simulink model "ASE_372K_FinalProj_AttD"  (R2018b)
settings: Solver=VariableStepAuto  StartTime=0.0  StopTime=5370  FixedStep=100  RelTol=1e-3
libraries: simulink x3, sharedtransform x3
settings Model: SimulationMode=accelerator  Creator=kenda  LastModifiedBy=kenda

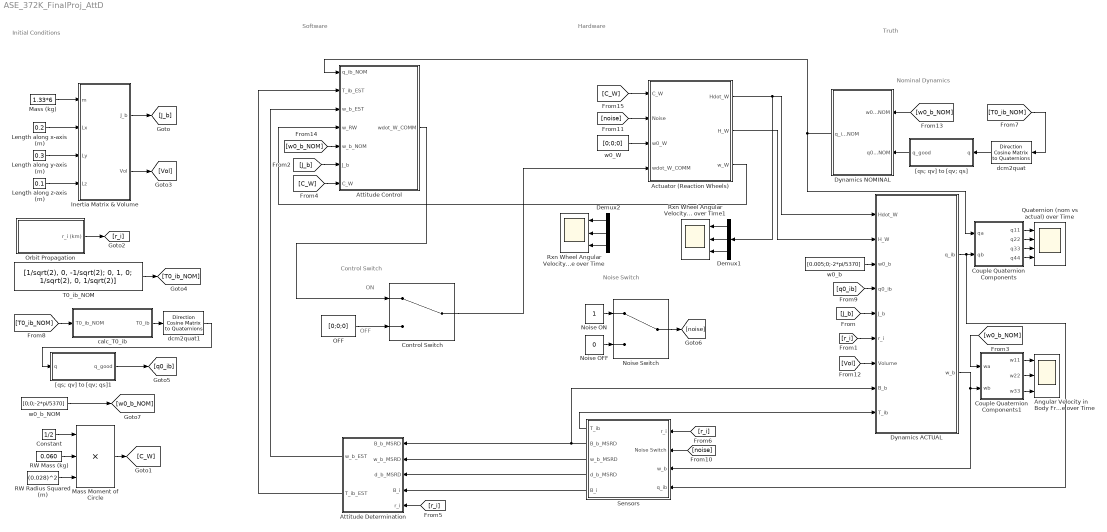
== system ASE_372K_FinalProj_AttD ==
  note: ON
  note: Truth
  note: Software
  note: Hardware
  note: Noise Switch
  note: OFF
  note: Control Switch
  note: Initial Conditions
  note: Nominal Dynamics
  Actuator (Reaction Wheels) : Subsystem
  Angular Velocity in Body Frame over Time : Scope  NumInputPorts=3
  Attitude Control : Subsystem
  Attitude Determination : Subsystem
  Constant : Constant  Value=1/2
  Control Switch : ManualSwitch
  Couple Quaternion Components : MATLAB Function  TreatAsAtomicUnit=on
  Couple Quaternion Components1 : MATLAB Function  TreatAsAtomicUnit=on
  Demux1 : Demux  Outputs=3
  Demux2 : Demux  Outputs=3
  Dynamics ACTUAL : Subsystem
  Dynamics NOMINAL : Subsystem
  Inertia Matrix & Volume : MATLAB Function  TreatAsAtomicUnit=on
  Length along x-axis (m) : Constant  Value=0.2
  Length along y-axis (m) : Constant  Value=0.3
  Length along z-axis (m) : Constant  Value=0.1
  Mass (kg) : Constant  Value=1.33*6
  Mass Moment of Circle : Product  Inputs=3
  Noise OFF : Constant  Value=0
  Noise ON : Constant
  Noise Switch : ManualSwitch
  OFF : Constant  Value=[0;0;0]
  Orbit Propagation : Subsystem
  Quaternion (nom vs actual) over Time : Scope  NumInputPorts=4
  RW Mass (kg) : Constant  Value=0.060
  RW Radius Squared (m) : Constant  Value=(0.028)^2
  Rxn Wheel Angular Velocity in Body Frame over Time : Scope  NumInputPorts=3
  Rxn Wheel Angular Velocity in Body Frame over Time1 : Scope  NumInputPorts=3
  Sensors : Subsystem
  T0_ib_NOM : Constant  Value=[1/sqrt(2), 0, -1/sqrt(2); 0, 1, 0; 1/sqrt(2), 0, 1/sqrt(2)]
  "[qs; qv] to [qv; qs]" : MATLAB Function  TreatAsAtomicUnit=on
  "[qs; qv] to [qv; qs]1" : MATLAB Function  TreatAsAtomicUnit=on
  calc_T0_ib : MATLAB Function  TreatAsAtomicUnit=on
  dcm2quat : sharedtransform/Direction Cosine Matrix  to Quaternions  aMode=0  action=None  tolerance=eps(2)
      settings: SourceProductName=Aerospace Blockset  SourceProductBaseCode=AE
  dcm2quat1 : sharedtransform/Direction Cosine Matrix  to Quaternions  aMode=0  action=None  tolerance=eps(2)
      settings: SourceProductName=Aerospace Blockset  SourceProductBaseCode=AE
  w0_W : Constant  Value=[0;0;0]
  w0_b : Constant  Value=[0.005;0;-2*pi/5370]
  w0_b_NOM : Constant  Value=[0;0;-2*pi/5370]
  wires:
  Dynamics ACTUAL/2(w_b) -> Couple Quaternion Components1/2(wb), Sensors/3(w_b)
  w0_W/1 -> Actuator (Reaction Wheels)/3(w0_W)
  w0_b/1 -> Dynamics ACTUAL/3(w0_b)
  [J_b] -> Dynamics ACTUAL/5(J_b)
  Actuator (Reaction Wheels)/2(H_W) -> Dynamics ACTUAL/2(H_W)
  [q0_ib] -> Dynamics ACTUAL/4(q0_ib)
  [C_W] -> Actuator (Reaction Wheels)/1(C_W)
  Actuator (Reaction Wheels)/1(Hdot_W) -> Demux1/1, Dynamics ACTUAL/1(Hdot_W)
  Sensors/3(w_b_MSRD) -> Attitude Determination/2(w_b_MSRD)
  Sensors/2(B_b_MSRD) -> Dynamics ACTUAL/8(B_b), Attitude Determination/1(B_b_MSRD)
  Dynamics ACTUAL/1(q_ib) -> Sensors/4(q_ib), Couple Quaternion Components/2(qb)
  [r_i] -> Attitude Determination/5(r_i)
  [r_i] -> Sensors/1(r_i)
  Actuator (Reaction Wheels)/3(w_W) -> Attitude Control/4(w_RW)
  Attitude Determination/1(w_b_EST) -> Attitude Control/3(w_b_EST)
  Attitude Determination/2(T_ib_EST) -> Attitude Control/2(T_ib_EST)
  Dynamics NOMINAL/1(q_ib_NOM) -> Couple Quaternion Components/1(qa), Attitude Control/1(q_ib_NOM)
  Attitude Control/1(wdot_W_COMM) -> Control Switch/1
  [J_b] -> Attitude Control/6(J_b)
  dcm2quat/1 -> "[qs; qv] to [qv; qs]"/1(q)
  [T0_ib_NOM] -> dcm2quat/1
  [T0_ib_NOM] -> calc_T0_ib/1(T0_ib_NOM)
  T0_ib_NOM/1 -> [T0_ib_NOM]
  dcm2quat1/1 -> "[qs; qv] to [qv; qs]1"/1(q)
  calc_T0_ib/1(T0_ib) -> dcm2quat1/1
  "[qs; qv] to [qv; qs]1"/1(q_good) -> [q0_ib]
  "[qs; qv] to [qv; qs]"/1(q_good) -> Dynamics NOMINAL/2(q0_ib_NOM)
  Noise Switch/1 -> [noise]
  Noise ON/1 -> Noise Switch/1
  Noise OFF/1 -> Noise Switch/2
  [noise] -> Sensors/2(Noise Switch)
  [noise] -> Actuator (Reaction Wheels)/2("Noise ")
  Control Switch/1 -> Actuator (Reaction Wheels)/4(wdot_W_COMM)
  Demux2/2 -> Rxn Wheel Angular Velocity in Body Frame over Time/2
  Demux2/1 -> Rxn Wheel Angular Velocity in Body Frame over Time/1
  Demux2/3 -> Rxn Wheel Angular Velocity in Body Frame over Time/3
  Orbit Propagation/1(r_i (km)) -> [r_i]
  [r_i] -> Dynamics ACTUAL/6(r_i)
  Mass (kg)/1 -> Inertia Matrix & Volume/1(m)
  Sensors/4(d_b_MSRD) -> Attitude Determination/3(d_b_MSRD)
  Sensors/5(B_i) -> Attitude Determination/4(B_i)
  Sensors/1(T_ib) -> Dynamics ACTUAL/9(T_ib)
  Inertia Matrix & Volume/2(Vol) -> [Vol]
  [Vol] -> Dynamics ACTUAL/7(Volume)
  w0_b_NOM/1 -> [w0_b_NOM]
  [w0_b_NOM] -> Dynamics NOMINAL/1(w0_b_NOM)
  [w0_b_NOM] -> Attitude Control/5(w_b_NOM)
  OFF/1 -> Control Switch/2
  [C_W] -> Attitude Control/7(C_W)
  Inertia Matrix & Volume/1(J_b) -> [J_b]
  Length along y-axis (m)/1 -> Inertia Matrix & Volume/3(Ly)
  Length along x-axis (m)/1 -> Inertia Matrix & Volume/2(Lx)
  Length along z-axis (m)/1 -> Inertia Matrix & Volume/4(Lz)
  Constant/1 -> Mass Moment of Circle/1
  RW Mass (kg)/1 -> Mass Moment of Circle/2
  RW Radius Squared (m)/1 -> Mass Moment of Circle/3
  Mass Moment of Circle/1 -> [C_W]
  Couple Quaternion Components/1(q11) -> Quaternion (nom vs actual) over Time/1
  Couple Quaternion Components/2(q22) -> Quaternion (nom vs actual) over Time/2
  Couple Quaternion Components/3(q33) -> Quaternion (nom vs actual) over Time/3
  Couple Quaternion Components/4(q44) -> Quaternion (nom vs actual) over Time/4
  Couple Quaternion Components1/1(w11) -> Angular Velocity in Body Frame over Time/1
  Couple Quaternion Components1/2(w22) -> Angular Velocity in Body Frame over Time/2
  Couple Quaternion Components1/3(w33) -> Angular Velocity in Body Frame over Time/3
  [w0_b_NOM] -> Couple Quaternion Components1/1(wa)
  Demux1/2 -> Rxn Wheel Angular Velocity in Body Frame over Time1/2
  Demux1/3 -> Rxn Wheel Angular Velocity in Body Frame over Time1/3
  Demux1/1 -> Rxn Wheel Angular Velocity in Body Frame over Time1/1

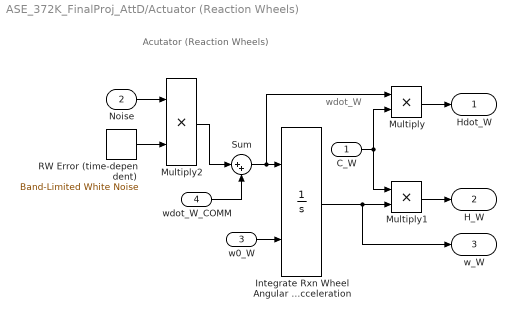
== system ASE_372K_FinalProj_AttD/Actuator (Reaction Wheels) ==
  note: wdot_W
  note: Acutator (Reaction Wheels)
  C_W : Inport
  "Noise " : Inport  Port=2
  w0_W : Inport  Port=3
  wdot_W_COMM : Inport  Port=4
  Integrate Rxn Wheel Angular Acceleration : Integrator  InitialConditionSource=external  ContinuousStateAttributes='ang_vel'
  Multiply : Product
  Multiply1 : Product
  Multiply2 : Product
  RW Error (time-dependent) : simulink/Sources/Band-Limited White Noise  Cov=1e-6*[1;1;1]  Ts=1  seed=[23341]
  Sum : Sum  Inputs=|++
  Hdot_W : Outport
  H_W : Outport  Port=2
  w_W : Outport  Port=3
  wires:
  w0_W/1 -> Integrate Rxn Wheel Angular Acceleration/2
  Sum/1 -> Multiply/1, Integrate Rxn Wheel Angular Acceleration/1
  RW Error (time-dependent)/1 -> Multiply2/2
  Multiply/1 -> Hdot_W/1
  C_W/1 -> Multiply1/1, Multiply/2
  Integrate Rxn Wheel Angular Acceleration/1 -> w_W/1, Multiply1/2
  Multiply1/1 -> H_W/1
  "Noise "/1 -> Multiply2/1
  Multiply2/1 -> Sum/1
  wdot_W_COMM/1 -> Sum/2

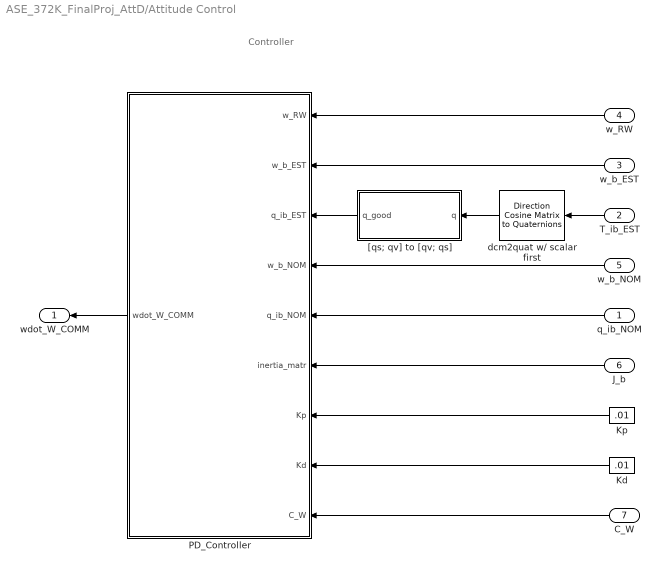
== system ASE_372K_FinalProj_AttD/Attitude Control ==
  note: Controller
  q_ib_NOM : Inport
  T_ib_EST : Inport  Port=2
  w_b_EST : Inport  Port=3
  w_RW : Inport  Port=4
  w_b_NOM : Inport  Port=5
  J_b : Inport  Port=6
  C_W : Inport  Port=7
  Kd : Constant  Value=.01
  Kp : Constant  Value=.01
  PD_Controller : MATLAB Function  TreatAsAtomicUnit=on
  "[qs; qv] to [qv; qs]" : MATLAB Function  TreatAsAtomicUnit=on
  dcm2quat w/ scalar first : sharedtransform/Direction Cosine Matrix  to Quaternions  aMode=0  action=None  tolerance=eps(2)
      settings: SourceProductName=Aerospace Blockset  SourceProductBaseCode=AE
  wdot_W_COMM : Outport
  wires:
  Kd/1 -> PD_Controller/8(Kd)
  w_b_NOM/1 -> PD_Controller/4(w_b_NOM)
  Kp/1 -> PD_Controller/7(Kp)
  J_b/1 -> PD_Controller/6(inertia_matr)
  PD_Controller/1(wdot_W_COMM) -> wdot_W_COMM/1
  C_W/1 -> PD_Controller/9(C_W)
  w_RW/1 -> PD_Controller/1(w_RW)
  w_b_EST/1 -> PD_Controller/2(w_b_EST)
  q_ib_NOM/1 -> PD_Controller/5(q_ib_NOM)
  T_ib_EST/1 -> dcm2quat w/ scalar first/1
  dcm2quat w/ scalar first/1 -> "[qs; qv] to [qv; qs]"/1(q)
  "[qs; qv] to [qv; qs]"/1(q_good) -> PD_Controller/3(q_ib_EST)

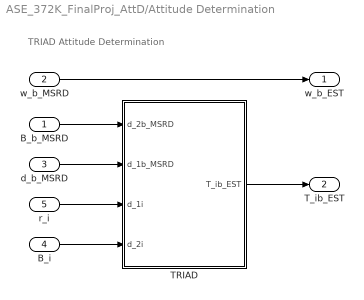
== system ASE_372K_FinalProj_AttD/Attitude Determination ==
  note: TRIAD Attitude Determination
  B_b_MSRD : Inport
  w_b_MSRD : Inport  Port=2
  d_b_MSRD : Inport  Port=3
  B_i : Inport  Port=4
  r_i : Inport  Port=5
  TRIAD : MATLAB Function  TreatAsAtomicUnit=on
  w_b_EST : Outport
  T_ib_EST : Outport  Port=2
  wires:
  w_b_MSRD/1 -> w_b_EST/1
  d_b_MSRD/1 -> TRIAD/2(d_1b_MSRD)
  B_b_MSRD/1 -> TRIAD/1(d_2b_MSRD)
  r_i/1 -> TRIAD/3(d_1i)
  B_i/1 -> TRIAD/4(d_2i)
  TRIAD/1(T_ib_EST) -> T_ib_EST/1

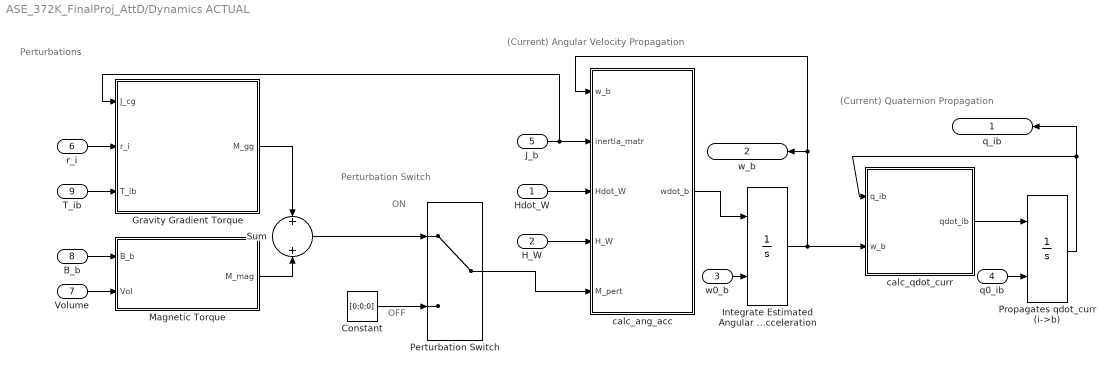
== system ASE_372K_FinalProj_AttD/Dynamics ACTUAL ==
  note: ON
  note: Perturbations
  note: (Current) Angular Velocity Propagation
  note: (Current) Quaternion Propagation
  note: OFF
  note: Perturbation Switch
  Hdot_W : Inport
  H_W : Inport  Port=2
  w0_b : Inport  Port=3
  q0_ib : Inport  Port=4
  J_b : Inport  Port=5
  r_i : Inport  Port=6
  Volume : Inport  Port=7
  B_b : Inport  Port=8
  T_ib : Inport  Port=9
  Constant : Constant  Value=[0;0;0]
  Gravity Gradient Torque : MATLAB Function  TreatAsAtomicUnit=on
  Integrate Estimated Angular Acceleration : Integrator  InitialConditionSource=external  ContinuousStateAttributes='ang_vel'
  Magnetic Torque : MATLAB Function  TreatAsAtomicUnit=on
  Perturbation Switch : ManualSwitch
  Propagates qdot_curr (i->b) : Integrator  InitialConditionSource=external  ContinuousStateAttributes='qdot_curr'
  Sum : Sum  Inputs=+||+
  calc_ang_acc : MATLAB Function  TreatAsAtomicUnit=on
  calc_qdot_curr : MATLAB Function  TreatAsAtomicUnit=on
  q_ib : Outport
  w_b : Outport  Port=2
  wires:
  w0_b/1 -> Integrate Estimated Angular Acceleration/2
  Integrate Estimated Angular Acceleration/1 -> w_b/1, calc_ang_acc/1(w_b), calc_qdot_curr/2(w_b)
  q0_ib/1 -> Propagates qdot_curr (i->b)/2
  calc_qdot_curr/1(qdot_ib) -> Propagates qdot_curr (i->b)/1
  Propagates qdot_curr (i->b)/1 -> calc_qdot_curr/1(q_ib), q_ib/1
  H_W/1 -> calc_ang_acc/4(H_W)
  Hdot_W/1 -> calc_ang_acc/3(Hdot_W)
  calc_ang_acc/1(wdot_b) -> Integrate Estimated Angular Acceleration/1
  r_i/1 -> Gravity Gradient Torque/2(r_i)
  J_b/1 -> Gravity Gradient Torque/1(J_cg), calc_ang_acc/2(inertia_matr)
  B_b/1 -> Magnetic Torque/1(B_b)
  Magnetic Torque/1(M_mag) -> Sum/2
  T_ib/1 -> Gravity Gradient Torque/3(T_ib)
  Gravity Gradient Torque/1(M_gg) -> Sum/1
  Volume/1 -> Magnetic Torque/2(Vol)
  Sum/1 -> Perturbation Switch/1
  Constant/1 -> Perturbation Switch/2
  Perturbation Switch/1 -> calc_ang_acc/5(M_pert)

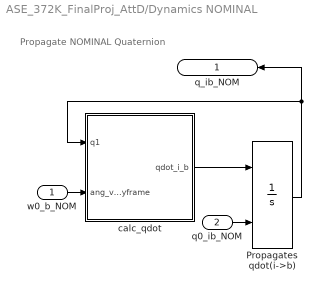
== system ASE_372K_FinalProj_AttD/Dynamics NOMINAL ==
  note: Propagate NOMINAL Quaternion
  w0_b_NOM : Inport
  q0_ib_NOM : Inport  Port=2
  Propagates qdot(i->b) : Integrator  InitialConditionSource=external  ContinuousStateAttributes='qdot_curr'
  calc_qdot : MATLAB Function  TreatAsAtomicUnit=on
  q_ib_NOM : Outport
  wires:
  q0_ib_NOM/1 -> Propagates qdot(i->b)/2
  Propagates qdot(i->b)/1 -> q_ib_NOM/1, calc_qdot/1(q1)
  calc_qdot/1(qdot_i_b) -> Propagates qdot(i->b)/1
  w0_b_NOM/1 -> calc_qdot/2(ang_vel_bodyframe)

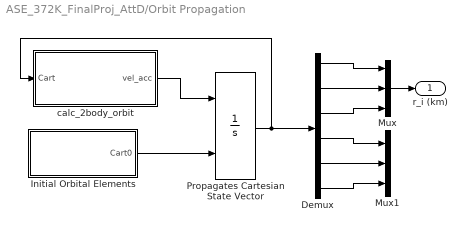
== system ASE_372K_FinalProj_AttD/Orbit Propagation ==
  Demux : Demux  Outputs=6
  Initial Orbital Elements : MATLAB Function  TreatAsAtomicUnit=on
  Mux : Mux  Inputs=3
  Mux1 : Mux  Inputs=3
  Propagates Cartesian State Vector : Integrator  InitialConditionSource=external  ContinuousStateAttributes='qdot_curr'
  calc_2body_orbit : MATLAB Function  TreatAsAtomicUnit=on
  r_i (km) : Outport
  wires:
  Initial Orbital Elements/1(Cart0) -> Propagates Cartesian State Vector/2
  calc_2body_orbit/1(vel_acc) -> Propagates Cartesian State Vector/1
  Propagates Cartesian State Vector/1 -> calc_2body_orbit/1(Cart), Demux/1
  Demux/3 -> Mux/3
  Demux/2 -> Mux/2
  Demux/1 -> Mux/1
  Demux/4 -> Mux1/1
  Demux/5 -> Mux1/2
  Demux/6 -> Mux1/3
  Mux/1 -> r_i (km)/1

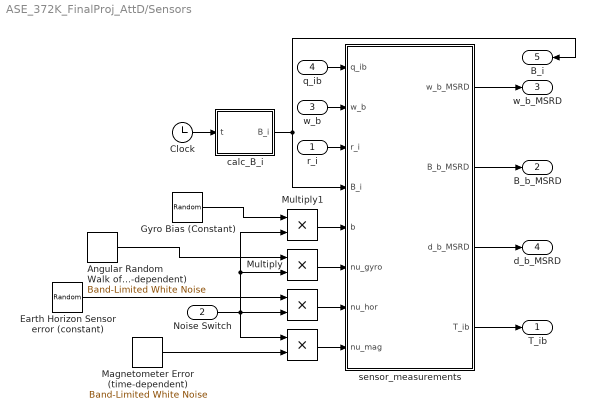
== system ASE_372K_FinalProj_AttD/Sensors ==
  r_i : Inport
  Noise Switch : Inport  Port=2
  w_b : Inport  Port=3
  q_ib : Inport  Port=4
  " " : Product
  "  " : Product
  Angular Random Walk of gyro (time-dependent) : simulink/Sources/Band-Limited White Noise  Cov=(0.3*pi/180)^2*[1;1;1]  Ts=1  seed=[23343]
  Clock : Clock
  Earth Horizon Sensor error (constant) : RandomNumber  Variance=(0.25*pi/180)^2  Seed=785
  Gyro Bias (Constant) : RandomNumber  Variance=(.01*pi/180)^2*[1;1;1]
  Magnetometer Error (time-dependent) : simulink/Sources/Band-Limited White Noise  Cov=(16e-9)^2*[1;1;1]  Ts=1  seed=[23343]
  Multiply : Product
  Multiply1 : Product
  calc_B_i : MATLAB Function  TreatAsAtomicUnit=on
  sensor_measurements : MATLAB Function  TreatAsAtomicUnit=on
  T_ib : Outport
  B_b_MSRD : Outport  Port=2
  w_b_MSRD : Outport  Port=3
  d_b_MSRD : Outport  Port=4
  B_i : Outport  Port=5
  wires:
  q_ib/1 -> sensor_measurements/1(q_ib)
  w_b/1 -> sensor_measurements/2(w_b)
  r_i/1 -> sensor_measurements/3(r_i)
  calc_B_i/1(B_i) -> sensor_measurements/4(B_i), B_i/1
  sensor_measurements/2(B_b_MSRD) -> B_b_MSRD/1
  sensor_measurements/3(d_b_MSRD) -> d_b_MSRD/1
  Clock/1 -> calc_B_i/1(t)
  Multiply/1 -> sensor_measurements/6(nu_gyro)
  Multiply1/1 -> sensor_measurements/5(b)
  Noise Switch/1 -> "  "/1, " "/2, Multiply1/2, Multiply/2
  sensor_measurements/1(w_b_MSRD) -> w_b_MSRD/1
  "  "/1 -> sensor_measurements/8(nu_mag)
  " "/1 -> sensor_measurements/7(nu_hor)
  sensor_measurements/4(T_ib) -> T_ib/1
  Gyro Bias (Constant)/1 -> Multiply1/1
  Magnetometer Error (time-dependent)/1 -> "  "/2
  Earth Horizon Sensor error (constant)/1 -> " "/1
  Angular Random Walk of gyro (time-dependent)/1 -> Multiply/1

== matlab function ASE_372K_FinalProj_AttD/Dynamics ACTUAL/calc_ang_acc ==
  data: w_b input; inertia_matr input; Hdot_W input; H_W input; M_pert input; wdot_b output
function wdot_b =...
    calc_ang_acc(w_b,inertia_matr,Hdot_W,H_W,M_pert)

% function returning angular acceleration of body axes wrt inertial axes in
% inertial frame
% % INPUTS
% w_b: 3x1 vec of ang vel of body wrt inertial in body frame
% M_pert: 3x1 vec of perturbation moments affecting attitude
% intertia_matr: 3x3 matrix of mass moments of inertia of a rigid body
% % OUTPUTS
% wdot_b: 3x1 vec of angular accel of body wrt inertial in bodyframe

% if exist('M_pert') == 0
%     M_pert = 0;
% end%if

% Shortening variable names for readability
w = w_b; % rad/s
J = inertia_matr;
Hdot = Hdot_W;
H = H_W;

% Calculating angular acceleration
wdot_b = J \ (-1*cross(w,J*w) - Hdot - cross(w,H) + M_pert); % rad/s^2

end%funciton

== matlab function ASE_372K_FinalProj_AttD/Dynamics ACTUAL/calc_qdot_curr ==
  data: q_ib input; w_b input; qdot_ib output
function qdot_ib = calc_qdot_ib(q_ib,w_b)

q2 = [w_b; 0]; % shortening variable name

% q1 is the current quaternion & q2 represents the quaternion for the new
% angular velocity

qdot_ib = 0.5 * quat_mult(q2,q_ib);

end

== matlab function ASE_372K_FinalProj_AttD/Orbit Propagation/Initial Orbital Elements ==
  data: Cart0 output
function Cart0 = KOE_0

% Orbital Constants
mu_earth = 398600.4415; % standard gravitation parameter of Earth (km^3/s^2)
R_Earth = 6378.1; % Radius of Earth (km)
alt = 406; % Altitude of s/c orbit (km)

% Keplerian Orbital Elements
sma = R_Earth + alt; % km
ecc = 0;
inc = 45*pi/180; % rads
raan = 90*pi/180; % rads
arg = -90*pi/180; % rads
tru = 0;
KOE0 = [sma; ecc; inc; raan; arg; tru];

w = sqrt(mu_earth/sma^3); % Orbital rotation rate (rad/s)
Period = 2*pi / w; % Orbital period (seconds)

% Function converting intial KOE to Cartesian state vector
[Cart0] = kep2cart_Whitbeck( mu_earth, KOE0 );

end%function

== matlab function ASE_372K_FinalProj_AttD/Attitude Control/[qs; qv] to [qv; qs] ==
  data: q input; q_good output
function q_good = flip_quat(q)

q_good = zeros(4,1);

q_good(1,1) = q(2);
q_good(2,1) = q(3);
q_good(3,1) = q(4);
q_good(4,1) = q(1);

end%function

== matlab function ASE_372K_FinalProj_AttD/Attitude Control/PD_Controller ==
  data: w_RW input; w_b_EST input; q_ib_EST input; w_b_NOM input; q_ib_NOM input; inertia_matr input; Kp input; Kd input; C_W input; wdot_W_COMM output
function wdot_W_COMM  = ...
    PD_controller(w_RW,w_b_EST,q_ib_EST,w_b_NOM,q_ib_NOM,inertia_matr,Kp,Kd,C_W)
% function calculating the commanded angular acceleration needed to correct
% the error & error rate between the estimated & nominal attitude of a rigid body.
%
% INPUTS
% % inertia_matr: inertia matrix of rigid body in body frame
% % Kp_gain: scalar, proportional gain
% % Kd_gain: scalar, derivative gain
%
% % OUTPUTS
% wdot_b_COMM: 3x1, commanded ang accel for RWs

J = inertia_matr;

wCur = w_b_EST;
wNom = w_b_NOM;
qCur = q_ib_EST;
qNom = q_ib_NOM;

% Conjugate nominal quaternion
qNomStar = quat_conjugate(qNom);

% Quaternion multiply to get quaternion control error, dq
dq = quat_mult(qCur,qNomStar);

% Calculate roll-pitch-yaw error angles vec
error = 2 * dq(1:3) ./ dq(4);

% difference in angular velocity btwn current & nominal
dw = wCur - wNom;

% skew-symmetric matrix representing wCur cross another vector
wX = skewSymMat(wCur);

% calculate roll-pitch-yaw error rate
error_rate = -wX * error + dw;

% Commanded angular acceleration
wdot_W_COMM = J*Kd/C_W*error + J*Kp/C_W*error_rate - cross(w_b_EST,w_RW);

end%function

== matlab function ASE_372K_FinalProj_AttD/Sensors/sensor_measurements ==
  data: q_ib input; w_b input; r_i input; B_i input; w_b_MSRD output; B_b_MSRD output; d_b_MSRD output; b input; nu_gyro input; nu_hor input; nu_mag input; T_ib output
function [w_b_MSRD, B_b_MSRD, d_b_MSRD, T_ib] = ...
    sensor_measurements(q_ib,w_b,r_i,B_i,b,nu_gyro,nu_hor,nu_mag)
% % INPUTS
% q_ib: 4x1, quaternion from inertial to body
% w_b: 3x1, ang vel of body wrt inertial in body frame
% r_i: 3x1, position in inertial frame
% b: 3x1, gyro bias
% nu_gyro: 3x1, random angular walk
% nu_mag: 3x1, magnetometer error
% nu_hor: 3x1, Earth Horizon error
% % OUTPUTS
% w_b_MSRD: 3x1, gyro measurement of ang vel of body wrt inertial in body frame
% B_b_MSRD: 3x1, magnetometer measurement
% d_b_MSRD: 3x1, Earth horizon sensor measurement

% Pre-calculations
qv = q_ib(1:3);
qs = q_ib(4);
qvx = skewSymMat(qv);
T_ib = eye(3,3) - 2*qs*qvx + 2*qvx^2;

% Getting measurements
w_b_MSRD = w_b + b + nu_gyro;
B_b_MSRD = T_ib * B_i + nu_mag;
d_b_MSRD = R3(nu_hor)*R1(nu_hor)*R3(nu_hor) * T_ib * - r_i/norm(r_i);

end %function

== matlab function ASE_372K_FinalProj_AttD/Sensors/calc_B_i ==
  data: t input; B_i output
function B_i = calc_B_i(t)

% Constants
mu = 3.986004418e14; % Standard Gravitational Parameter of Earth (m^3/s^2)
B0 = 3.12e-5; % mean value of Earth magnetic field at equator (Tesla)
Re = 6378137; % Earth radius at equator (meters)

% Orbit parameters
rho = 6600e3; % orbit radius, const bc circular orbit(meters)
w = sqrt(mu/rho^3); % rad/s

% z-component of unit vec in inertial frame
i_zi = [0; 0; 1];

% Position in inertial frame (meters)
r_i_vec = rho/sqrt(2) * [-cos(w*t); sqrt(2)*sin(w*t); cos(w*t)];

% Latitude (rad)
lat = asin(r_i_vec(3)/rho);

% Magnetic field of Earth as dipole
B_n = B0 * (Re/rho)^3 * [cos(lat); 0; -2*sin(lat)];

% Transformation Components
n_zi = -r_i_vec / rho;
n_yi = cross(n_zi, i_zi) / norm(cross(n_zi, i_zi));
n_xi = cross(n_yi, n_zi);
T_in = [n_xi'; n_yi'; n_zi'];

% Magnetic field in inertial frame
B_i = T_in' * B_n;

end%function

== matlab function ASE_372K_FinalProj_AttD/Attitude Determination/TRIAD ==
  data: d_2b_MSRD input; T_ib_EST output; d_1b_MSRD input; d_1i input; d_2i input
function T_ib_EST = triad(d_2b_MSRD, d_1b_MSRD, d_1i, d_2i)
% % INPUTS
% d_1b: 3x1, most accurate body measurement (from Earth Horizon sensor)
% d_2b: 3x1, less accurate body measurement (from Magnetometer body-frame)
% d_1i: 3x1, inertial position (given) (r_i)
% d_2i: 3x1, inertial position (from Magnetometer inertial-frame) (B_i)

x_b = d_1b_MSRD / norm(d_1b_MSRD);
z_b = cross(x_b,d_2b_MSRD) / norm(cross(x_b,d_2b_MSRD));
y_b = cross(z_b,x_b);% / norm(cross(z_b,x_b));

x_i = -d_1i / norm(d_1i);
z_i = cross(x_i,d_2i) / norm(cross(x_i,d_2i));
y_i = cross(z_i,x_i);% / norm(cross(z_i,x_i));

T_ib_EST = [x_b y_b z_b] * [x_i y_i z_i]';

end%function

== matlab function ASE_372K_FinalProj_AttD/[qs; qv] to [qv; qs] ==
  data: q input; q_good output
function q_good = flip_quat(q)

q_good = zeros(4,1);

q_good(1,1) = q(2);
q_good(2,1) = q(3);
q_good(3,1) = q(4);
q_good(4,1) = q(1);

end%function

== matlab function ASE_372K_FinalProj_AttD/Orbit Propagation/calc_2body_orbit ==
  data: Cart input; vel_acc output
function vel_acc = calc_2body_orbit(Cart)
% Propagates Carteisan Orbital Elements using 2-Body Dynamics
% INPUT:
% % Cart: 6x1, Cartesian State st Cart(1:3) is the position & Cart(4:6) is
% % velocity
% OUTPUT:
% % vel_acc: 6x1, Cartesian velocity (1:3) & acceleration (4:6)

 % standard gravitation parameter of Earth
 mu_earth = 398600.4415; % km^3/s^2

% Cartesian velocity (km/s) (1:3) & acceleration (km/s^2) (4:6)
vel_acc = [Cart(4:6); -mu_earth .* Cart(1:3) ./ (norm(Cart(1:3))^3)];

end

== matlab function ASE_372K_FinalProj_AttD/calc_T0_ib ==
  data: T0_ib_NOM input; T0_ib output
function T0_ib = calc_T0_ib(T0_ib_NOM)
% functiong getting actual initial DCM from inertial to body

T0_ib = R2(2*pi/180) * T0_ib_NOM;

end%function

== matlab function ASE_372K_FinalProj_AttD/Dynamics NOMINAL/calc_qdot ==
  data: q1 input; ang_vel_bodyframe input; qdot_i_b output
function qdot_i_b = calc_qdot(q1,ang_vel_bodyframe)

qdot_i_b = calc_qdot_i_b(ang_vel_bodyframe,q1);

end

== matlab function ASE_372K_FinalProj_AttD/[qs; qv] to [qv; qs]1 ==
  data: q input; q_good output
function q_good = flip_quat(q)

q_good = zeros(4,1);

q_good(1,1) = q(2);
q_good(2,1) = q(3);
q_good(3,1) = q(4);
q_good(4,1) = q(1);

end%function

== matlab function ASE_372K_FinalProj_AttD/Dynamics ACTUAL/Gravity Gradient Torque ==
  data: J_cg input; r_i input; M_gg output; T_ib input
function M_gg  = calc_M_gg(J_cg,r_i,T_ib)
% function calculating the perturbation torque due to gravity-gradient of
% the spacecraft (s/c)'s center of gravity (cg)
% INPUTS:
% % r_i: 3x1, position of s/c's cg in inertial frame (m)
% % J_cg: 3x3, inertia matrix (kg-m^2)
% % db: 3x1, pointing direction of body
% OUTPUT:
% % M_gg: 3x1, perturabtion torque due to gravity gradient (N-m)

mu_Earth = 398600.4415; % standard gravitation parameter of Earth (km^3/s^2)

% Transform s/c's cg into body frame
d_i = -r_i / norm(r_i);
d_b = T_ib * d_i;

% Orbital Angular Velocity of s/c around Earth
w_orb = sqrt(mu_Earth / norm(r_i)^3);

% perturabtion torque due to gravity gradient (N-m)
M_gg = 3 * w_orb^2  * cross(d_b,J_cg*d_b);

end%function

== matlab function ASE_372K_FinalProj_AttD/Dynamics ACTUAL/Magnetic Torque ==
  data: B_b input; M_mag output; Vol input
function M_mag = calc_M_mag(B_b,Vol)
% function calculating the torque on a spacecraft due to magnetic fields
% INPUT:
% % B_b: 3x1, components of Earth's magentic field in body frame (Tesla)
% % Dims: 3x1, [Length; Width; Depth] (m)
% OUTPUT:
% % M_mag: 3x1, perturbation torques due to magnetic fields

% Constant of s/c
M = 0.9; % Magnetization Parameter of s/c (Ampere-meter^2) (varies 0.1-0.9)

% Magnetic field of the spacecraft pointing thru body y-axis (along
% velocity direction)
Bsat = Vol * M * [0;1;0]; % Tesla

% Torque due to Magnetic fields interacting
M_mag = cross(Bsat,B_b); % N-m

end%function

== matlab function ASE_372K_FinalProj_AttD/Inertia Matrix & Volume ==
  data: m input; Lx input; J_b output; Ly input; Lz input; Vol output
function [J_b,Vol] = calc_J_b(m,Lx,Ly,Lz)
% Mass Moment of Inertia Matrix of a rectangular prism
% % INPUTS:
% m: mass of s/c (kg)
% Lx: width (along x-axis) of rect prism (m)
% Ly: length (along y-axis) of rect prism (m)
% Lz: depth (along z-axis) of rect prism (m)
% % OUTPUTS:
% J_b: 3x3, inertia matrix for rect prism

% Volume of s/c
Vol = Lx*Ly*Lz; % m^3

% Moments of Inertia along the principal axes
Ixx = 1/12 * m * (Ly^2 + Lz^2); % kg-m^2
Iyy = 1/12 * m * (Lx^2 + Lz^2); % kg-m^2
Izz = 1/12 * m * (Lx^2 + Ly^2); % kg-m^2

% Mass moment of Inertia (kg-m^2)
J_b = [Ixx 0 0;
    0 Iyy 0;
    0 0 Izz];

end%function

== matlab function ASE_372K_FinalProj_AttD/Couple Quaternion Components ==
  data: qa input; q11 output; qb input; q22 output; q33 output; q44 output
function [q11, q22, q33, q44] = quatCouple(qa,qb)
% function coupling the components of 2 quaternions into 4 vectors

q11 = [qa(1); qb(1)];
q22 = [qa(2); qb(2)];
q33 = [qa(3); qb(3)];
q44 = [qa(4); qb(4)];

end%function

== matlab function ASE_372K_FinalProj_AttD/Couple Quaternion Components1 ==
  data: wa input; w11 output; wb input; w22 output; w33 output
function [w11, w22, w33] = quatCouple(wa,wb)
% function coupling the components of 2 angular vels into 3 couples

w11 = [wa(1); wb(1)];
w22 = [wa(2); wb(2)];
w33 = [wa(3); wb(3)];

end%function
